simulink model "BPSK_DemodManchester"  (R2013a)
settings: Solver=FixedStepDiscrete  SolverMode=SingleTasking  StartTime=0.0  StopTime=10000/2400  FixedStep=1/480e3  RelTol=1e-3
undefined symbols (not defined in the file or in its folder): DiscIntNeverNeededParam
libraries: dspsigops x6, commsynccomp2 x4, dsparch4 x3, simulink x2, simulink_extras x1, commchan3 x1, commsink2 x1, commrflib2 x1, commrandsrc2 x1
settings Model: Creator=tibbs2010  LastModifiedBy=Cedric
settings DataIOCC: SignalLoggingSaveFormat=ModelDataLogs
settings DebuggingCC: MultiTaskDSMMsg=warning  MultiTaskCondExecSysMsg=none  StrictBusMsg=None
settings RTWCC: IncludeERTFirstTime=on

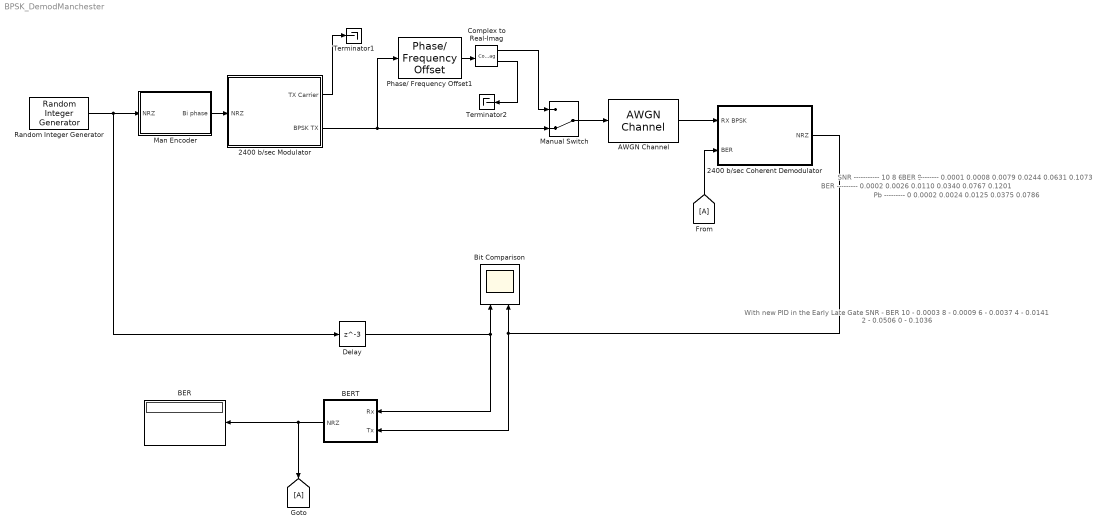
== system BPSK_DemodManchester ==
  note: With new PID in the Early Late Gate
      |
      | SNR    - BER
      | 10   -     0.0003
      | 8 -         0.0009
      | 6 -         0.0037
      | 4 -         0.0141
      | 2 -         0.0506
      | 0 -         0.1036
  note: BER
      | ---------
      | 0.0002
      | 0.0026
      | 0.0110
      | 0.0340
      | 0.0767
      | 0.1201
  note: SNR
      | -----------
      |    10
      |      8
      |      6
      |      4
      |      2
      |      0
  note: Pb
      | ---------
      | 0
      | 0.0002
      | 0.0024
      | 0.0125
      | 0.0375
      | 0.0786
  note: BER
      | ---------
      | 0.0001
      | 0.0008
      | 0.0079
      | 0.0244
      | 0.0631
      | 0.1073
  " 2400 b/sec Coherent Demodulator" : Subsystem
  2400 b/sec Modulator : Subsystem
  AWGN Channel : commchan3/AWGN Channel  InputProcessing=Columns as channels (frame based)  seed=randseed  noiseMode="Signal to noise ratio  (Eb/No)"  EbNodB=10  EsNodB=10  SNRdB=10  bitsPerSym=1  Ps=12.5  Tsym=1/2400  variance=1
  BER : Display
  BERT : Subsystem
  Bit Comparison : Scope  NumInputPorts=2
      settings: TimeRange=0.008608695652173926  YMin=-0.5~-0.5  YMax=1.5~1.5
  Complex to Real-Imag : ComplexToRealImag
  Delay : Delay  DelayLength=3  SampleTime=1/1200
  Man Encoder : Subsystem
  Manual Switch : ManualSwitch  CurrentSetting=0
  Phase/ Frequency Offset1 : commrflib2/Phase// Frequency Offset  phaseOffset=30  freqPort=off  freqOffset=0
  Random Integer Generator : commrandsrc2/Random Integer Generator  mul=2  seed=randseed  Ts=1/1200  frameBased=off  sampPerFrame=1  orient=off  outDataType=double
  Terminator1 : Terminator
  Terminator2 : Terminator
  wires:
  2400 b/sec Modulator/2(BPSK TX) -> Manual Switch/2, Phase/ Frequency Offset1/1
  Manual Switch/1 -> AWGN Channel/1
  Phase/ Frequency Offset1/1 -> Complex to Real-Imag/1
  Complex to Real-Imag/1 -> Manual Switch/1
  AWGN Channel/1 -> " 2400 b/sec Coherent Demodulator"/1(RX BPSK)
  " 2400 b/sec Coherent Demodulator"/1(NRZ) -> Bit Comparison/2, BERT/2(Tx)
  Man Encoder/1(Bi phase) -> 2400 b/sec Modulator/1(NRZ)
  2400 b/sec Modulator/1(TX Carrier) -> Terminator1/1
  BERT/1(NRZ) -> BER/1, [A]
  [A] -> " 2400 b/sec Coherent Demodulator"/2("BER ")
  Delay/1 -> BERT/1(Rx), Bit Comparison/1
  Random Integer Generator/1 -> Delay/1, Man Encoder/1(NRZ)
  Complex to Real-Imag/2 -> Terminator2/1

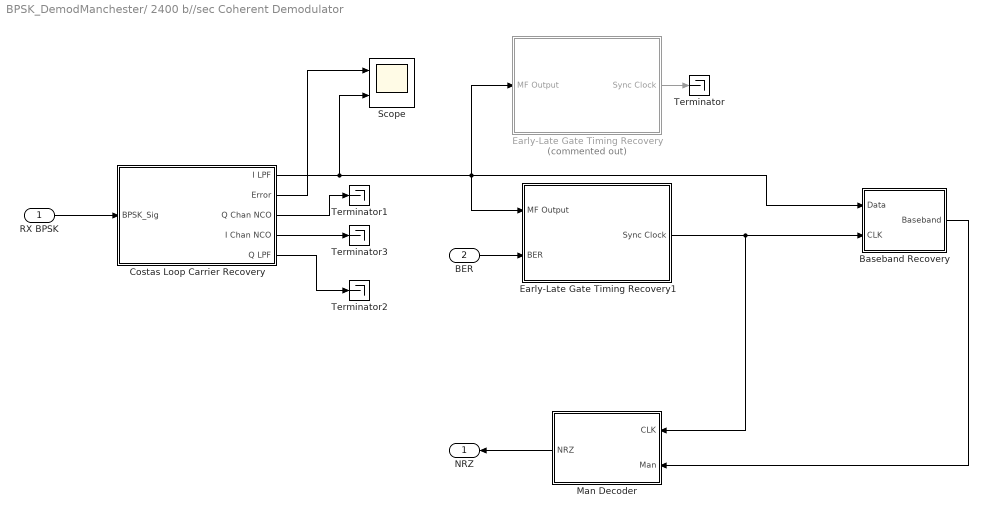
== system BPSK_DemodManchester/ 2400 b//sec Coherent Demodulator ==
  RX BPSK : Inport
  "BER " : Inport  Port=2
  Baseband Recovery : Subsystem
  Costas Loop Carrier Recovery : Subsystem
  Early-Late Gate Timing Recovery : Subsystem  Commented=on
  Early-Late Gate Timing Recovery1 : Subsystem
  Man Decoder : Subsystem
  Scope : Scope  NumInputPorts=2
      settings: TimeRange=0.0403041825095057  YMin=-30~-12.5  YMax=30~12.5
  Terminator{,1..3} (4 alike) : Terminator
  NRZ : Outport
  wires:
  RX BPSK/1 -> Costas Loop Carrier Recovery/1(BPSK_Sig)
  Costas Loop Carrier Recovery/1(I LPF) -> Scope/2, Early-Late Gate Timing Recovery/1(MF Output), Baseband Recovery/1(Data), Early-Late Gate Timing Recovery1/1(MF Output)
  Costas Loop Carrier Recovery/2(Error) -> Scope/1
  Early-Late Gate Timing Recovery1/1(Sync Clock) -> Man Decoder/1(CLK), Baseband Recovery/2(CLK)
  Baseband Recovery/1(Baseband) -> Man Decoder/2(Man)
  "BER "/1 -> Early-Late Gate Timing Recovery1/2("BER ")
  Early-Late Gate Timing Recovery/1(Sync Clock) -> Terminator/1
  Costas Loop Carrier Recovery/3(Q Chan NCO) -> Terminator1/1
  Costas Loop Carrier Recovery/5(Q LPF) -> Terminator2/1
  Costas Loop Carrier Recovery/4(I Chan NCO) -> Terminator3/1
  Man Decoder/1(NRZ) -> NRZ/1

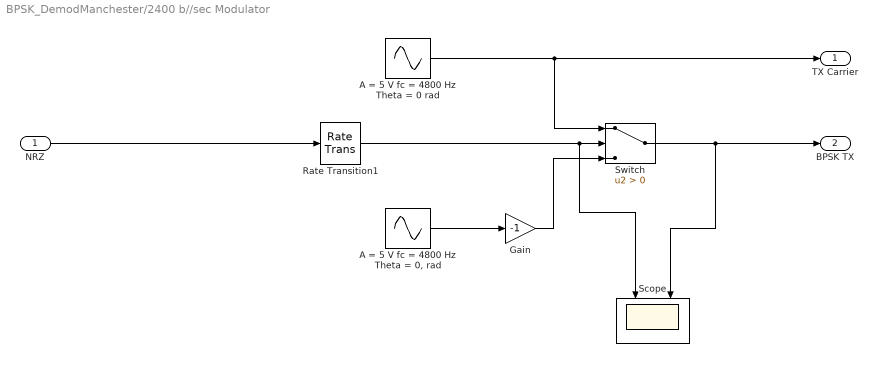
== system BPSK_DemodManchester/2400 b//sec Modulator ==
  NRZ : Inport
  A = 5 V fc = 4800 Hz Theta = 0 rad : Sin  Amplitude=5  Frequency=2*pi*4800  Phase=pi/2  SampleTime=1/480e3
  "A = 5 V fc = 4800 Hz Theta = 0, rad" : Sin  Amplitude=5  Frequency=2*pi*4800  Phase=pi/2  Samples=100  SampleTime=1/480e3  Offset=pi
  Gain : Gain  Gain=-1
  Rate Transition1 : RateTransition  OutPortSampleTime=1/480e3
  Scope : Scope  NumInputPorts=2
      settings: TimeRange=0.06  YMin=-1000~-0.5  YMax=1000~1.5  SaveName=ScopeData2
  Switch : Switch  Criteria=u2 > Threshold
  TX Carrier : Outport
  BPSK TX : Outport  Port=2
  wires:
  A = 5 V fc = 4800 Hz Theta = 0 rad/1 -> TX Carrier/1, Switch/1
  "A = 5 V fc = 4800 Hz Theta = 0, rad"/1 -> Gain/1
  Gain/1 -> Switch/3
  NRZ/1 -> Rate Transition1/1
  Switch/1 -> BPSK TX/1, Scope/2
  Rate Transition1/1 -> Scope/1, Switch/2

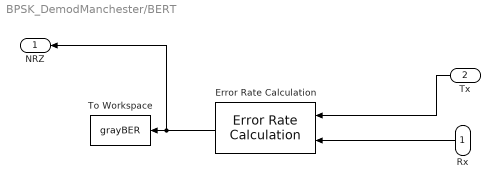
== system BPSK_DemodManchester/BERT ==
  Rx : Inport
  Tx : Inport  Port=2
  Error Rate Calculation : commsink2/Error Rate Calculation  N=0  st_delay=0  cp_mode=Entire frame  subframe=[]  PMode=Port  WsName=grayBER  RsMode2=off  stop=off  numErr=maxNumErrs  maxBits=maxNumBits
  To Workspace : ToWorkspace  VariableName=grayBER  SampleTime=-1  SaveFormat=Timeseries
      settings: MaxDataPoints=1
  NRZ : Outport
  wires:
  Error Rate Calculation/1 -> NRZ/1, To Workspace/1
  Rx/1 -> Error Rate Calculation/2
  Tx/1 -> Error Rate Calculation/1

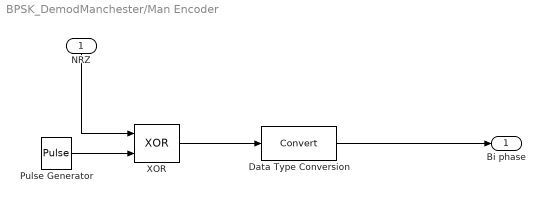
== system BPSK_DemodManchester/Man Encoder ==
  NRZ : Inport
  Data Type Conversion : DataTypeConversion
  Pulse Generator : DiscretePulseGenerator  SampleTime=1/(1200*2)
  XOR : Logic  Operator=XOR  IconShape=distinctive  AllPortsSameDT=off  OutDataTypeStr=boolean
  Bi phase : Outport
  wires:
  XOR/1 -> Data Type Conversion/1
  Pulse Generator/1 -> XOR/2
  NRZ/1 -> XOR/1
  Data Type Conversion/1 -> Bi phase/1

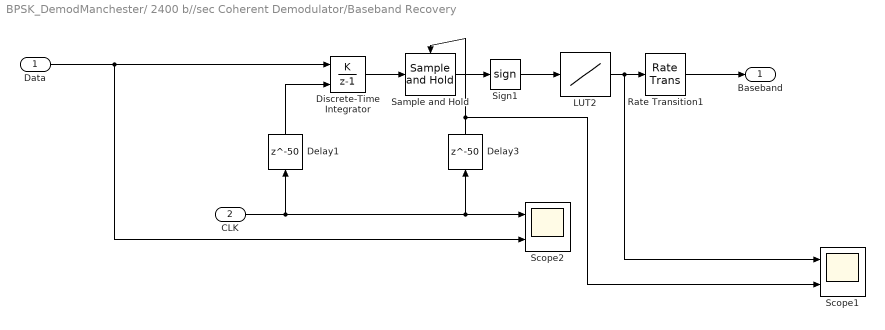
== system BPSK_DemodManchester/ 2400 b//sec Coherent Demodulator/Baseband Recovery ==
  Data : Inport
  CLK : Inport  Port=2
  Delay1 : Delay  DelayLength=50  InitialCondition=0
  Delay3 : Delay  DelayLength=50  InitialCondition=0
  Discrete-Time Integrator : DiscreteIntegrator  IntegratorMethod=Accumulation: Forward Euler  ExternalReset=rising  SampleTime=1/480e3  ICPrevOutput=DiscIntNeverNeededParam  ICPrevScaledInput=DiscIntNeverNeededParam
  LUT2 : Lookup_n-D  NumberOfTableDimensions=1  BreakpointsForDimension1=[-1 0 1]  Table=[0 0 1]  RndMeth=Simplest  InputSameDT=on
  Rate Transition1 : RateTransition  OutPortSampleTime=1/2400
  Sample and Hold : dspsigops/Sample and Hold  trig=Rising edge  initCond=0  latchinput=on
  Scope1 : Scope  NumInputPorts=2
      settings: TimeRange=0.01093750000000002  YMin=-0.5~-0.5  YMax=1.5~1.5  SaveName=ScopeData4
  Scope2 : Scope  NumInputPorts=2
      settings: TimeRange=0.01093750000000002  YMin=-0.5~-0.5  YMax=1.5~1.5  SaveName=ScopeData9
  Sign1 : Signum
  Baseband : Outport
  wires:
  Sign1/1 -> LUT2/1
  Sample and Hold/1 -> Sign1/1
  Rate Transition1/1 -> Baseband/1
  Discrete-Time Integrator/1 -> Sample and Hold/1
  Delay1/1 -> Discrete-Time Integrator/2
  CLK/1 -> Scope2/1, Delay3/1, Delay1/1
  Delay3/1 -> Sample and Hold/Trigger, Scope1/2
  LUT2/1 -> Scope1/1, Rate Transition1/1
  Data/1 -> Scope2/2, Discrete-Time Integrator/1

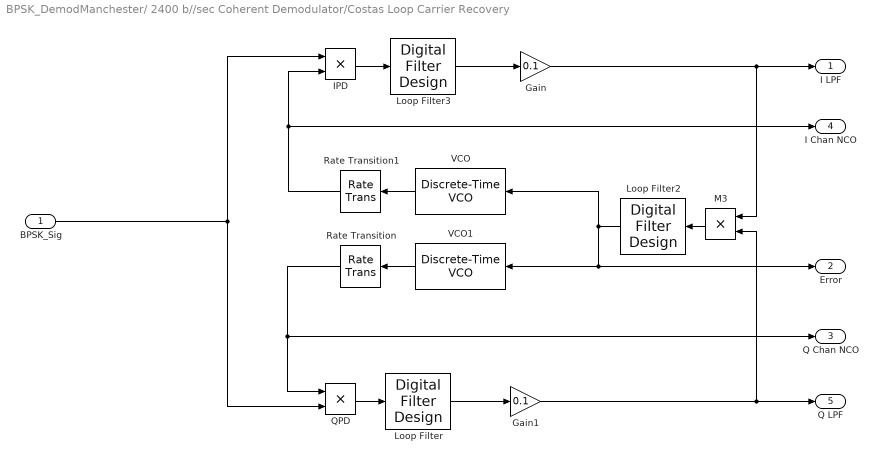
== system BPSK_DemodManchester/ 2400 b//sec Coherent Demodulator/Costas Loop Carrier Recovery ==
  BPSK_Sig : Inport
  Gain : Gain  Gain=0.1
  Gain1 : Gain  Gain=0.1
  IPD : Product  SampleTime=1/480e3
  Loop Filter : dsparch4/Digital Filter Design  mwdsp_browser_bugfix_var=off
  Loop Filter2 : dsparch4/Digital Filter Design  mwdsp_browser_bugfix_var=off
  Loop Filter3 : dsparch4/Digital Filter Design  mwdsp_browser_bugfix_var=off
  M3 : Product  SampleTime=1/480e3
  QPD : Product  SampleTime=1/480e3
  Rate Transition : RateTransition  OutPortSampleTime=1/480e3
  Rate Transition1 : RateTransition  OutPortSampleTime=1/480e3
  VCO : commsynccomp2/Discrete-Time VCO  Ac=5  Fc=4800  Kc=0.5  Ph=0  ts=1/480e3
  VCO1 : commsynccomp2/Discrete-Time VCO  Ac=5  Fc=4800  Kc=0.5  Ph=pi/2  ts=1/480e3
  I LPF : Outport
  Error : Outport  Port=2
  Q Chan NCO : Outport  Port=3
  I Chan NCO : Outport  Port=4
  Q LPF : Outport  Port=5
  wires:
  VCO/1 -> Rate Transition1/1
  VCO1/1 -> Rate Transition/1
  Rate Transition/1 -> QPD/1, Q Chan NCO/1
  Rate Transition1/1 -> IPD/2, I Chan NCO/1
  QPD/1 -> Loop Filter/1
  IPD/1 -> Loop Filter3/1
  BPSK_Sig/1 -> IPD/1, QPD/2
  Loop Filter/1 -> Gain1/1
  Loop Filter3/1 -> Gain/1
  M3/1 -> Loop Filter2/1
  Loop Filter2/1 -> VCO/1, Error/1, VCO1/1
  Gain/1 -> I LPF/1, M3/1
  Gain1/1 -> Q LPF/1, M3/2

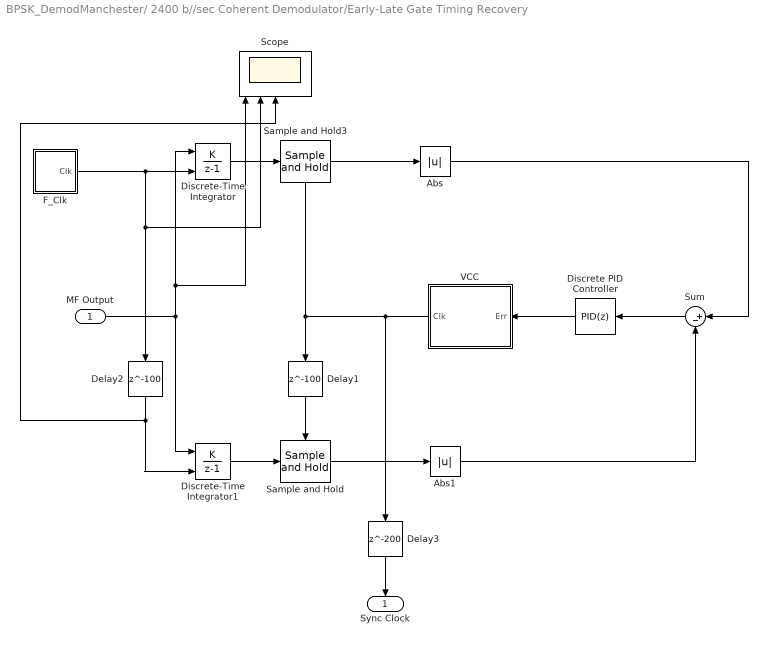
== system BPSK_DemodManchester/ 2400 b//sec Coherent Demodulator/Early-Late Gate Timing Recovery ==
  MF Output : Inport
  Abs : Abs
  Abs1 : Abs
  Delay1 : Delay  DelayLength=100  InitialCondition=0
  Delay2 : Delay  DelayLength=100  InitialCondition=0
  Delay3 : Delay  DelayLength=200  InitialCondition=0
  Discrete PID Controller : simulink/Continuous/PID Controller  Controller=PID  TimeDomain=Discrete-time  SampleTime=1/480e3  IntegratorMethod=Forward Euler  FilterMethod=Forward Euler  Form=Parallel  P=0.1  I=0.01  D=0  N=0  InitialConditionSource=internal  InitialConditionForIntegrator=0  InitialConditionForFilter=0  ExternalReset=none  LimitOutput=off  UpperSaturationLimit=inf  LowerSaturationLimit=-inf  LinearizeAsGain=off  AntiWindupMode=none  Kb=1  TrackingMode=off  Kt=1  PParamMin=[]  PParamMax=[]  IParamMin=[]  IParamMax=[]  DParamMin=[]  DParamMax=[]  NParamMin=[]  NParamMax=[]  KbParamMin=[]  KbParamMax=[]  KtParamMin=[]  KtParamMax=[]  POutMin=[]  POutMax=[]  IOutMin=[]  IOutMax=[]  DOutMin=[]  DOutMax=[]  NOutMin=[]  NOutMax=[]  KbOutMin=[]  KbOutMax=[]  KtOutMin=[]  KtOutMax=[]  IntegratorOutMin=[]  IntegratorOutMax=[]  FilterOutMin=[]  FilterOutMax=[]  SumOutMin=[]  SumOutMax=[]  SumI1OutMin=[]  SumI1OutMax=[]  SumI2OutMin=[]  SumI2OutMax=[]  SumI3OutMin=[]  SumI3OutMax=[]  SumDOutMin=[]  SumDOutMax=[]  SaturationOutMin=[]  SaturationOutMax=[]  IntegratorContinuousStateAttributes=''  IntegratorStateMustResolveToSignalObject=off  IntegratorRTWStateStorageClass=Auto  FilterContinuousStateAttributes=''  FilterStateMustResolveToSignalObject=off  FilterRTWStateStorageClass=Auto
  Discrete-Time Integrator : DiscreteIntegrator  IntegratorMethod=Accumulation: Forward Euler  ExternalReset=rising  SampleTime=1/480e3  ICPrevOutput=DiscIntNeverNeededParam  ICPrevScaledInput=DiscIntNeverNeededParam
  Discrete-Time Integrator1 : DiscreteIntegrator  IntegratorMethod=Accumulation: Forward Euler  ExternalReset=rising  SampleTime=1/480e3  ICPrevOutput=DiscIntNeverNeededParam  ICPrevScaledInput=DiscIntNeverNeededParam
  F_Clk : Subsystem
  Sample and Hold : dspsigops/Sample and Hold  trig=Rising edge  initCond=0  latchinput=off
  Sample and Hold3 : dspsigops/Sample and Hold  trig=Rising edge  initCond=0  latchinput=off
  Scope : Scope  NumInputPorts=5
      settings: TimeRange=0.06  YMin=110~-0.5~-0.5~-0.5~-200  YMax=160~1.5~1.5~1.5~200  SaveName=ScopeData3
  Sum : Sum  Inputs=|+-
  VCC : Subsystem
  Sync Clock : Outport
  wires:
  Abs1/1 -> Sum/2
  Sample and Hold/1 -> Abs1/1
  Sample and Hold3/1 -> Abs/1
  Sum/1 -> Discrete PID Controller/1
  VCC/1(Clk) -> Delay3/1, Delay1/1, Sample and Hold3/Trigger
  MF Output/1 -> Scope/1, Discrete-Time Integrator/1, Discrete-Time Integrator1/1
  Discrete-Time Integrator/1 -> Sample and Hold3/1
  Discrete-Time Integrator1/1 -> Sample and Hold/1
  Delay2/1 -> Scope/3, Discrete-Time Integrator1/2
  Delay1/1 -> Sample and Hold/Trigger
  Delay3/1 -> Sync Clock/1
  F_Clk/1(Clk) -> Scope/2, Delay2/1, Discrete-Time Integrator/2
  Discrete PID Controller/1 -> VCC/1(Err)
  Abs/1 -> Sum/1

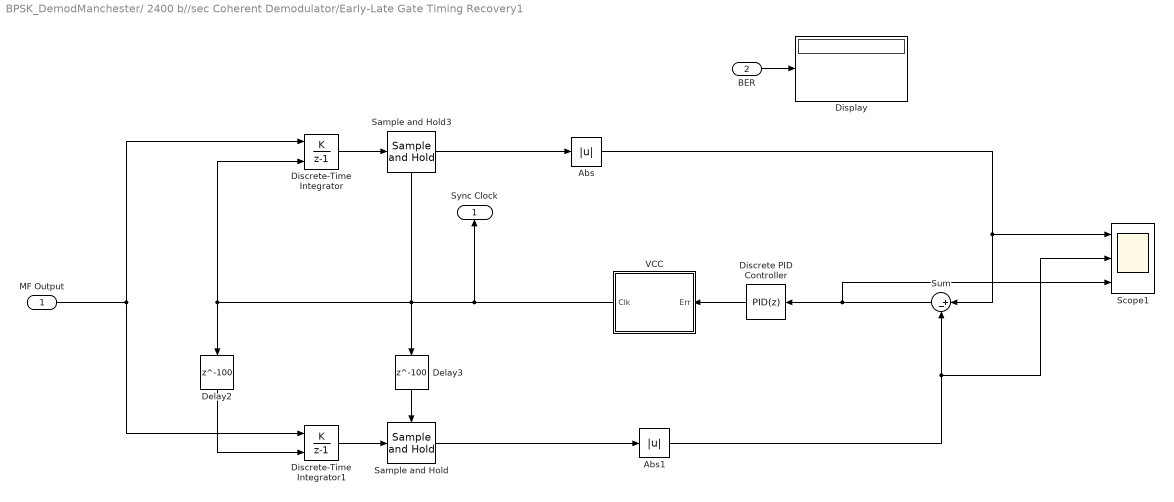
== system BPSK_DemodManchester/ 2400 b//sec Coherent Demodulator/Early-Late Gate Timing Recovery1 ==
  MF Output : Inport
  "BER " : Inport  Port=2
  Abs : Abs
  Abs1 : Abs
  Delay2 : Delay  DelayLength=100  InitialCondition=0
  Delay3 : Delay  DelayLength=100  InitialCondition=0
  Discrete PID Controller : simulink/Continuous/PID Controller  Controller=PID  TimeDomain=Discrete-time  SampleTime=1/480e3  IntegratorMethod=Forward Euler  FilterMethod=Forward Euler  Form=Parallel  P=0.01  I=0.1  D=0.0009  N=1  InitialConditionSource=internal  InitialConditionForIntegrator=0  InitialConditionForFilter=0  ExternalReset=none  LimitOutput=off  UpperSaturationLimit=inf  LowerSaturationLimit=-inf  LinearizeAsGain=off  AntiWindupMode=none  Kb=1  TrackingMode=off  Kt=1  PParamMin=[]  PParamMax=[]  IParamMin=[]  IParamMax=[]  DParamMin=[]  DParamMax=[]  NParamMin=[]  NParamMax=[]  KbParamMin=[]  KbParamMax=[]  KtParamMin=[]  KtParamMax=[]  POutMin=[]  POutMax=[]  IOutMin=[]  IOutMax=[]  DOutMin=[]  DOutMax=[]  NOutMin=[]  NOutMax=[]  KbOutMin=[]  KbOutMax=[]  KtOutMin=[]  KtOutMax=[]  IntegratorOutMin=[]  IntegratorOutMax=[]  FilterOutMin=[]  FilterOutMax=[]  SumOutMin=[]  SumOutMax=[]  SumI1OutMin=[]  SumI1OutMax=[]  SumI2OutMin=[]  SumI2OutMax=[]  SumI3OutMin=[]  SumI3OutMax=[]  SumDOutMin=[]  SumDOutMax=[]  SaturationOutMin=[]  SaturationOutMax=[]  IntegratorContinuousStateAttributes=''  IntegratorStateMustResolveToSignalObject=off  IntegratorRTWStateStorageClass=Auto  FilterContinuousStateAttributes=''  FilterStateMustResolveToSignalObject=off  FilterRTWStateStorageClass=Auto
  Discrete-Time Integrator : DiscreteIntegrator  IntegratorMethod=Accumulation: Forward Euler  ExternalReset=rising  SampleTime=1/480e3  ICPrevOutput=DiscIntNeverNeededParam  ICPrevScaledInput=DiscIntNeverNeededParam
  Discrete-Time Integrator1 : DiscreteIntegrator  IntegratorMethod=Accumulation: Forward Euler  ExternalReset=rising  SampleTime=1/480e3  ICPrevOutput=DiscIntNeverNeededParam  ICPrevScaledInput=DiscIntNeverNeededParam
  Display : Display
  Sample and Hold : dspsigops/Sample and Hold  trig=Rising edge  initCond=0  latchinput=on
  Sample and Hold3 : dspsigops/Sample and Hold  trig=Rising edge  initCond=0  latchinput=on
  Scope1 : Scope  NumInputPorts=3
      settings: TimeRange=0.208333  YMin=0~0~-250  YMax=400~400~300  SaveName=ScopeData5
  Sum : Sum  Inputs=|+-
  VCC : Subsystem
  Sync Clock : Outport
  wires:
  Abs1/1 -> Sum/2, Scope1/2
  Sample and Hold/1 -> Abs1/1
  Discrete-Time Integrator/1 -> Sample and Hold3/1
  Discrete-Time Integrator1/1 -> Sample and Hold/1
  MF Output/1 -> Discrete-Time Integrator/1, Discrete-Time Integrator1/1
  Discrete PID Controller/1 -> VCC/1(Err)
  Abs/1 -> Sum/1, Scope1/1
  Sample and Hold3/1 -> Abs/1
  Delay3/1 -> Sample and Hold/Trigger
  Delay2/1 -> Discrete-Time Integrator1/2
  VCC/1(Clk) -> Delay3/1, Sample and Hold3/Trigger, Discrete-Time Integrator/2, Delay2/1, Sync Clock/1
  "BER "/1 -> Display/1
  Sum/1 -> Discrete PID Controller/1, Scope1/3

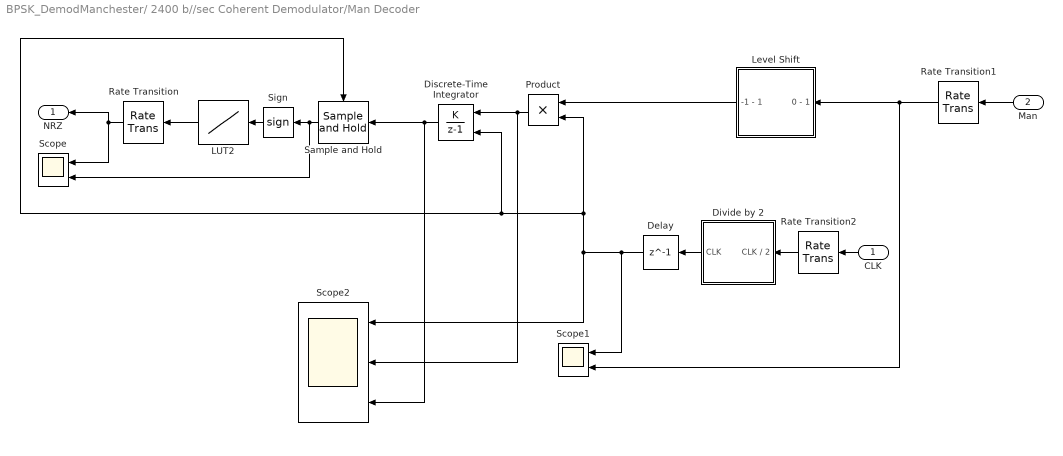
== system BPSK_DemodManchester/ 2400 b//sec Coherent Demodulator/Man Decoder ==
  CLK : Inport
  Man : Inport  Port=2
  Delay : Delay  DelayLength=1
  Discrete-Time Integrator : DiscreteIntegrator  IntegratorMethod=Accumulation: Forward Euler  ExternalReset=rising  SampleTime=1/(1200*10)  ICPrevOutput=DiscIntNeverNeededParam  ICPrevScaledInput=DiscIntNeverNeededParam
  Divide by 2 : Subsystem
  LUT2 : Lookup_n-D  NumberOfTableDimensions=1  BreakpointsForDimension1=[-1 0 1]  Table=[0 0 1]  RndMeth=Simplest  InputSameDT=on
  Level Shift : Subsystem
  Product : Product
  Rate Transition : RateTransition  OutPortSampleTime=1/1200
  Rate Transition1 : RateTransition  OutPortSampleTime=1/(1200*10)
  Rate Transition2 : RateTransition  OutPortSampleTime=1/(1200*10)
  Sample and Hold : dspsigops/Sample and Hold  trig=Falling edge  initCond=0  latchinput=off
  Scope : Scope  NumInputPorts=2
      settings: YMin=-5~-5  YMax=5~5  SaveName=ScopeData6
  Scope1 : Scope  NumInputPorts=2
      settings: TimeRange=0.007187739463601533  YMin=0~0  YMax=1~1  SaveName=ScopeData7
  Scope2 : Scope  NumInputPorts=3
      settings: YMin=-5~-5~-5  YMax=5~5~5  SaveName=ScopeData8
  Sign : Signum
  NRZ : Outport
  wires:
  CLK/1 -> Rate Transition2/1
  Product/1 -> Scope2/2, Discrete-Time Integrator/1
  Discrete-Time Integrator/1 -> Scope2/3, Sample and Hold/1
  Man/1 -> Rate Transition1/1
  Sample and Hold/1 -> Scope/2, Sign/1
  Sign/1 -> LUT2/1
  LUT2/1 -> Rate Transition/1
  Divide by 2/1(CLK) -> Delay/1
  Level Shift/1(-1 - 1) -> Product/1
  Rate Transition/1 -> Scope/1, NRZ/1
  Rate Transition1/1 -> Scope1/2, Level Shift/1(0 - 1)
  Rate Transition2/1 -> Divide by 2/1(CLK / 2)
  Delay/1 -> Product/2, Sample and Hold/Trigger, Discrete-Time Integrator/2, Scope2/1, Scope1/1

== system BPSK_DemodManchester/ 2400 b//sec Coherent Demodulator/Early-Late Gate Timing Recovery/F_Clk ==
  " " : DataTypeConversion  OutDataTypeStr=boolean
  Pulse Generator : DiscretePulseGenerator  PulseType=Time based  Amplitude=5  Period=1/2400  PulseWidth=50  SampleTime=1/480e3
  Clk : Outport
  wires:
  " "/1 -> Clk/1
  Pulse Generator/1 -> " "/1

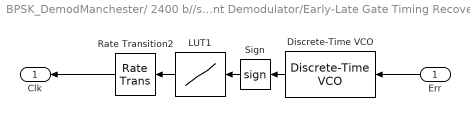
== system BPSK_DemodManchester/ 2400 b//sec Coherent Demodulator/Early-Late Gate Timing Recovery/VCC ==
  Err : Inport
  Discrete-Time VCO : commsynccomp2/Discrete-Time VCO  Ac=1  Fc=2400  Kc=1  Ph=1  ts=1/480e3
  LUT1 : Lookup_n-D  NumberOfTableDimensions=1  BreakpointsForDimension1=[-1 0 1]  Table=[0 0 1]  RndMeth=Simplest  InputSameDT=on
  Rate Transition2 : RateTransition  OutPortSampleTime=1/480e3
  Sign : Signum
  Clk : Outport
  wires:
  Discrete-Time VCO/1 -> Sign/1
  Err/1 -> Discrete-Time VCO/1
  LUT1/1 -> Rate Transition2/1
  Rate Transition2/1 -> Clk/1
  Sign/1 -> LUT1/1

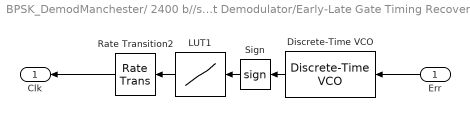
== system BPSK_DemodManchester/ 2400 b//sec Coherent Demodulator/Early-Late Gate Timing Recovery1/VCC ==
  Err : Inport
  Discrete-Time VCO : commsynccomp2/Discrete-Time VCO  Ac=1  Fc=2400  Kc=1  Ph=0  ts=1/480e3
  LUT1 : Lookup_n-D  NumberOfTableDimensions=1  BreakpointsForDimension1=[-1 0 1]  Table=[0 0 1]  RndMeth=Simplest  InputSameDT=on
  Rate Transition2 : RateTransition  OutPortSampleTime=1/480e3
  Sign : Signum
  Clk : Outport
  wires:
  Discrete-Time VCO/1 -> Sign/1
  Err/1 -> Discrete-Time VCO/1
  LUT1/1 -> Rate Transition2/1
  Rate Transition2/1 -> Clk/1
  Sign/1 -> LUT1/1

== system BPSK_DemodManchester/ 2400 b//sec Coherent Demodulator/Man Decoder/Divide by 2 ==
  CLK / 2 : Inport
  Constant1 : Constant
  D Flip-Flop : simulink_extras/Flip Flops/D Flip-Flop
  CLK : Outport
  wires:
  D Flip-Flop/1 -> CLK/1
  D Flip-Flop/2 -> D Flip-Flop/1
  Constant1/1 -> D Flip-Flop/3
  CLK / 2/1 -> D Flip-Flop/2

== system BPSK_DemodManchester/ 2400 b//sec Coherent Demodulator/Man Decoder/Level Shift ==
  0 - 1 : Inport
  Constant : Constant  Value=-0.5  SampleTime=1/(1200*10)
  Gain : Gain  Gain=2  SampleTime=1/(1200*10)
  Sum : Sum  Inputs=|++
  -1 - 1 : Outport
  wires:
  Sum/1 -> Gain/1
  Gain/1 -> -1 - 1/1
  Constant/1 -> Sum/2
  0 - 1/1 -> Sum/1
